simulink model "Satellte_Communications_System_TDMA"  (R2019b)
settings: Solver=ode45  StartTime=0.0  StopTime=inf  RelTol=1e-3  EnableMultiTasking=on
undefined symbols (not defined in the file): magnitude
libraries: dspstat3 x8, rfmathmodels1 x5, commrflib2 x4, commdigbbndpm3 x4, commfilt2 x4, dspsigattribs x4, dspmathops x4, dsparch4 x3, commrandsrc2 x2, commcnvcod2 x2, commsink2 x2, commutil2 x2
settings Model: Creator=123  LastModifiedBy=Steve
settings DataIOCC: LimitDataPoints=on  SaveFormat=Array  ReturnWorkspaceOutputs=off
settings OptimizationCC: LifeSpan=inf
settings DebuggingCC: SolverPrmCheckMsg=warning  SFUnexpectedBacktrackingDiag=warning  SFNoUnconditionalDefaultTransitionDiag=warning  SFExecutionAtInitializationDiag=none  ArithmeticOperatorsInVariantConditions=warning
settings HardwareCC: ProdBitPerPointer=32  ProdBitPerSizeT=32  ProdBitPerPtrDiffT=32  ProdLargestAtomicFloat=None  ProdIntDivRoundTo=Undefined  ProdEndianess=Unspecified  ProdWordSize=32  ProdHWDeviceType=32-bit Generic
settings ModelReferenceCC: PropagateSignalLabelsOutOfModel=off
settings SFSimCC: SimUseLocalCustomCode=off  CustomCodeUndefinedFunction=UseInterfaceOnly
settings RTWCC: RTWUseLocalCustomCode=off
settings CodeAppCC: StateflowObjectComments=on
settings GRTTargetCC: TargetLangStandard=C89/C90 (ANSI)  GeneratePreprocessorConditionals=Disable all
settings ConfigComp: CovMetricSettings=dw  CovHtmlReporting=on  CovSaveCumulativeToWorkspaceVar=on  CovSaveSingleToWorkspaceVar=on  CovExternalEMLEnable=off  CovSFcnEnable=off

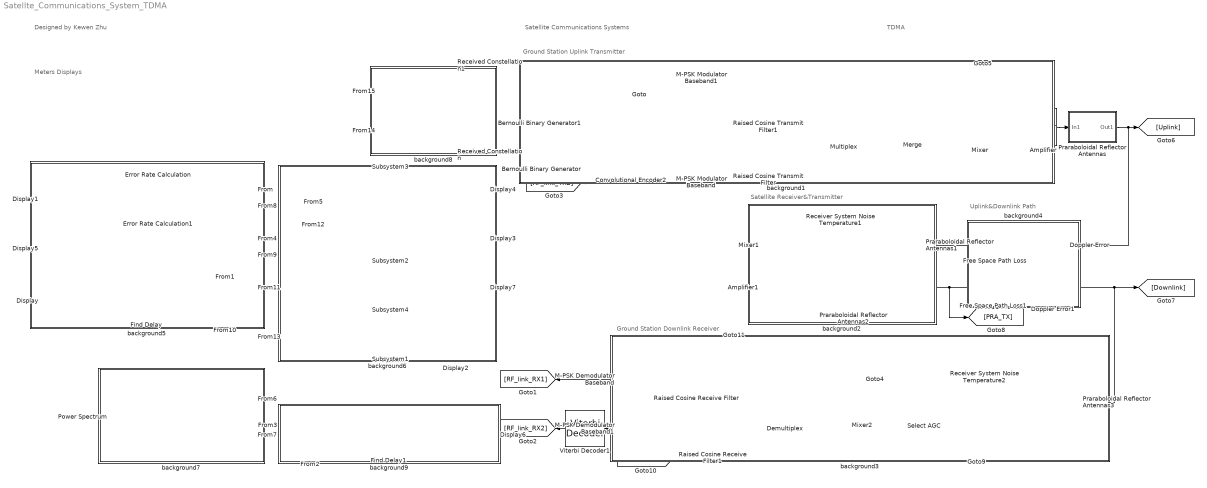
== system Satellte_Communications_System_TDMA ==
  note: Satellite Communications Systems
  note: Ground Station Uplink Transmitter
  note: Satellite Receiver&Transmitter
  note: Ground Station Downlink Receiver
  note: Uplink&Downlink Path
  note: Meters Displays
  note: Designed by Kewen Zhu
  note: TDMA
  Amplifier : rfmathmodels1/Amplifier  model_select=Saleh model  linGaindB=70  GindB=-21  iip3=30  am2pm=10  PwrAMPMStart=10  PwrAMPMEnd=inf  amam=[2.1587 1.1517]  ampm=[4.0033 9.1040]  x=[8.1081 1.5413 6.5202 -0.0718]  y=[4.6645 2.0965 10.88 -0.003]  p=0.5  GoutdB=70  vsat=1  method_select=Noise temperature  ntemp=0  nfigure=3.01  nfactor=2  seed=67987
      settings: SourceProductName=RF Blockset  SourceProductBaseCode=RB
  Amplifier1 : rfmathmodels1/Amplifier  model_select=Saleh model  linGaindB=84  GindB=-21  iip3=30  am2pm=10  PwrAMPMStart=10  PwrAMPMEnd=inf  amam=[2.1587 1.1517]  ampm=[4.0033 9.1040]  x=[8.1081 1.5413 6.5202 -0.0718]  y=[4.6645 2.0965 10.88 -0.003]  p=0.5  GoutdB=70  vsat=1  method_select=Noise temperature  ntemp=0  nfigure=3.01  nfactor=2  seed=67987
      settings: SourceProductName=RF Blockset  SourceProductBaseCode=RB
  Bernoulli Binary Generator : commrandsrc2/Bernoulli Binary Generator  P=0.5  seed=61  Ts=1/32000  frameBased=on  sampPerFrame=5100  orient=off  outDataType=double
      settings: SourceProductName=Communications Toolbox  SourceProductBaseCode=CM
  Bernoulli Binary Generator1 : commrandsrc2/Bernoulli Binary Generator  P=0.5  seed=61  Ts=1/64000  frameBased=on  sampPerFrame=10200  orient=off  outDataType=double
      settings: SourceProductName=Communications Toolbox  SourceProductBaseCode=CM
  Convolutional Encoder2 : commcnvcod2/Convolutional Encoder  trellis=poly2trellis(7, [171 133])  opMode=Continuous  DelayedResetAction=off  hasIniStPort=off  hasFinStPort=off  usePuncVector=off  punctureVector=[1; 1; 0; 1; 0; 1]  reset=Unused parameter value
      settings: SourceProductName=Communications Toolbox  SourceProductBaseCode=CM
  Demultiplex : Subsystem
  Display{,1..7} (8 alike) : Display
  Doppler Error : commrflib2/Phase// Frequency Offset  phaseOffset=0  freqPort=off  freqOffset=paramRFSatLink.DoppOffset
      settings: SourceProductName=Communications Toolbox
  Doppler Error1 : commrflib2/Phase// Frequency Offset  phaseOffset=0  freqPort=off  freqOffset=paramRFSatLink.DoppOffset
      settings: SourceProductName=Communications Toolbox
  Error Rate Calculation : commsink2/Error Rate Calculation  N=16  st_delay=0  cp_mode=Entire frame  subframe=[]  PMode=Port  WsName=ErrorVec  RsMode2=off  stop=off  numErr=100  maxBits=1e6
      settings: SourceProductName=Communications Toolbox
  Error Rate Calculation1 : commsink2/Error Rate Calculation  N=42  st_delay=0  cp_mode=Entire frame  subframe=[]  PMode=Port  WsName=ErrorVec  RsMode2=off  stop=off  numErr=100  maxBits=1e6
      settings: SourceProductName=Communications Toolbox
  Find Delay : commutil2/Find Delay  corrLength=200  chgSigOP=off  stopUpdate=off  numConstDelay=3
      settings: SourceProductName=Communications Toolbox  SourceProductBaseCode=CM
  Find Delay1 : commutil2/Find Delay  corrLength=200  chgSigOP=off  stopUpdate=off  numConstDelay=3
      settings: SourceProductName=Communications Toolbox  SourceProductBaseCode=CM
  Free Space Path Loss : commrflib2/Free Space Path Loss  mode=Distance and Frequency  dB=199  d=36000  fc=6000
      settings: SourceProductName=Communications Toolbox  SourceProductBaseCode=CM
  Free Space Path Loss1 : commrflib2/Free Space Path Loss  mode=Distance and Frequency  dB=196  d=36000  fc=4000
      settings: SourceProductName=Communications Toolbox  SourceProductBaseCode=CM
  M-PSK Demodulator Baseband : commdigbbndpm3/M-PSK Demodulator Baseband  M=4  OutType=Bit  DecType=Hard decision  VarSource=Dialog  Variance=1  Dec=Gray  Mapping=[0:7]  Ph=pi/4  outDtype1=Inherit via internal rule  outDtype2=Inherit via internal rule  derotateFactorWordLen=16  derotateFactorDataTypeStr=Inherit: Same word length as input  derotateFactorLastDataTypeStr=Inherit: Same word length as input
      settings: SourceProductName=Communications Toolbox
  M-PSK Demodulator Baseband1 : commdigbbndpm3/M-PSK Demodulator Baseband  M=4  OutType=Bit  DecType=Hard decision  VarSource=Dialog  Variance=1  Dec=Gray  Mapping=[0:7]  Ph=pi/4  outDtype1=Inherit via internal rule  outDtype2=Inherit via internal rule  derotateFactorWordLen=16  derotateFactorDataTypeStr=Inherit: Same word length as input  derotateFactorLastDataTypeStr=Inherit: Same word length as input
      settings: SourceProductName=Communications Toolbox
  M-PSK Modulator Baseband : commdigbbndpm3/M-PSK Modulator Baseband  M=4  InType=Bit  Enc=Gray  Mapping=[0:7]  Ph=pi/4  outDtype=double  outWordLen=16  outUDDataType=sfix(16)  outFracLenMode=Best precision  outFracLen=15  outDataTypeStr=double  outLastDataTypeStr=double
      settings: SourceProductName=Communications Toolbox
  M-PSK Modulator Baseband1 : commdigbbndpm3/M-PSK Modulator Baseband  M=4  InType=Bit  Enc=Gray  Mapping=[0:7]  Ph=pi/4  outDtype=double  outWordLen=16  outUDDataType=sfix(16)  outFracLenMode=Best precision  outFracLen=15  outDataTypeStr=double  outLastDataTypeStr=double
      settings: SourceProductName=Communications Toolbox
  Merge : Merge
  Mixer : rfmathmodels1/Mixer  gain=0  PhNs=-500  Fo=4e9  seed=2137  loss=0
      settings: SourceProductName=RF Blockset  SourceProductBaseCode=RB
  Mixer1 : rfmathmodels1/Mixer  gain=0  PhNs=-500  Fo=4e9  seed=2137  loss=0
      settings: SourceProductName=RF Blockset  SourceProductBaseCode=RB
  Mixer2 : rfmathmodels1/Mixer  gain=0  PhNs=-500  Fo=6e9  seed=2137  loss=0
      settings: SourceProductName=RF Blockset  SourceProductBaseCode=RB
  Multiplex : Subsystem
  Power Spectrum : Subsystem  TreatAsAtomicUnit=on
      mask Display: disp('Power\nSpectrum')
  Praraboloidal Reflector Antennas : Subsystem  mask(RF Transmit Antennas){f=6, D=15, g=0.6}
      mask prompts: f "Transmit Frequency(GHz)"; D "Antennas Caliber/Diameter(m)"; g "Gain factor(less than 1)"
      mask help:
      | Based on the Paraboloidal Reflector Antennas formula ,Gain factor is
      | G=(pi*D*f/c).^2*g
      mask init:
      | if isempty(f|D|g)
      |   gain= 0;
      |   s  = ['dB Gain'];
      | else
      |   f=f*10.^9;w=(3*10.^8)/f;
      |   G=(((pi*D/w).^2)*g).^0.5; 
      |   temp=((pi*D/w).^2)*g;
      |   gain=10*log10(temp);
      |   if (isscalar(f|D|g))
      |     s = sprintf('%g dB\n(%g)',gain,temp);
      |   else
      |     s = ['dB Gain'];
      |   end
      | end
      mask Display: fprintf(s)
  Praraboloidal Reflector Antennas1 : Subsystem  mask(RF Transmit Antennas){f=6, D=0.14, g=0.7}
      mask prompts: f "Transmit Frequency(GHz)"; D "Antennas Caliber/Diameter(m)"; g "Gain factor(less than 1)"
      mask help:
      | Based on the Paraboloidal Reflector Antennas formula ,Gain factor is
      | G=(pi*D*f/c).^2*g
      mask init: same as Satellte_Communications_System_TDMA/Praraboloidal Reflector Antennas
      mask Display: fprintf(s)
  Praraboloidal Reflector Antennas2 : Subsystem  mask(RF Transmit Antennas){f=4, D=0.4, g=0.7}
      mask prompts: f "Transmit Frequency(GHz)"; D "Antennas Caliber/Diameter(m)"; g "Gain factor(less than 1)"
      mask help:
      | Based on the Paraboloidal Reflector Antennas formula ,Gain factor is
      | G=(pi*D*f/c).^2*g
      mask init: same as Satellte_Communications_System_TDMA/Praraboloidal Reflector Antennas
      mask Display: fprintf(s)
  Praraboloidal Reflector Antennas3 : Subsystem  mask(RF Transmit Antennas){f=4, D=4.5, g=0.82}
      mask prompts: f "Transmit Frequency(GHz)"; D "Antennas Caliber/Diameter(m)"; g "Gain factor(less than 1)"
      mask help:
      | Based on the Paraboloidal Reflector Antennas formula ,Gain factor is
      | G=(pi*D*f/c).^2*g
      mask init: same as Satellte_Communications_System_TDMA/Praraboloidal Reflector Antennas
      mask Display: fprintf(s)
  Raised Cosine Receive Filter : commfilt2/Raised Cosine Receive Filter  filtType=Square root  R=0.2  filtSpan=8  N=8  downFactor=8  downOffset=0  filterGain=1  InputProcessing=Columns as channels (frame based)  RateOptions=Enforce single-rate processing  framing=Mute  checkCoeff=off  variableName=rcRxFilt  currentFiltSpan=8  D=(8)/2  inputOffset=0  sampMode=Mute  saveAsFlag=0  rateMode=Downsampling  checkGain=Normalized  launchFVT=on  roundingMode=Floor  overflowMode=off  coeffDataTypeStr=Inherit: Same word length as input  coeffMin=[]  coeffMax=[]  coeffLastDataTypeStr=Inherit: Same word length as input  accumDataTypeStr=Inherit: Same as product output  accumLastDataTypeStr=Inherit: Same as product output  outputDataTypeStr=Inherit: Same as accumulator  outputMin=[]  outputMax=[]  outputLastDataTypeStr=Inherit: Same as accumulator
      settings: SourceProductName=Communications Toolbox
  Raised Cosine Receive Filter1 : commfilt2/Raised Cosine Receive Filter  filtType=Square root  R=0.2  filtSpan=8  N=8  downFactor=8  downOffset=0  filterGain=1  InputProcessing=Columns as channels (frame based)  RateOptions=Enforce single-rate processing  framing=Mute  checkCoeff=off  variableName=rcRxFilt1  currentFiltSpan=8  D=(8)/2  inputOffset=0  sampMode=Mute  saveAsFlag=0  rateMode=Downsampling  checkGain=Normalized  launchFVT=on  roundingMode=Floor  overflowMode=off  coeffDataTypeStr=Inherit: Same word length as input  coeffMin=[]  coeffMax=[]  coeffLastDataTypeStr=Inherit: Same word length as input  accumDataTypeStr=Inherit: Same as product output  accumLastDataTypeStr=Inherit: Same as product output  outputDataTypeStr=Inherit: Same as accumulator  outputMin=[]  outputMax=[]  outputLastDataTypeStr=Inherit: Same as accumulator
      settings: SourceProductName=Communications Toolbox
  Raised Cosine Transmit Filter : commfilt2/Raised Cosine Transmit Filter  filtType=Square root  R=0.2  filtSpan=8  N=8  filterGain=1  InputProcessing=Columns as channels (frame based)  RateOptions=Enforce single-rate processing  framing=Mute  checkCoeff=off  variableName=rcTxFilt  checkGain=Normalized  sampMode=Mute  saveAsFlag=0  currentFiltSpan=8  D=(8)/2  launchFVT=on  roundingMode=Floor  overflowMode=off  coeffDataTypeStr=Inherit: Same word length as input  coeffMin=[]  coeffMax=[]  coeffLastDataTypeStr=Inherit: Same word length as input  outputDataTypeStr=Inherit: Same as accumulator  outputMin=[]  outputMax=[]  outputLastDataTypeStr=Inherit: Same as accumulator
      settings: SourceProductName=Communications Toolbox
  Raised Cosine Transmit Filter1 : commfilt2/Raised Cosine Transmit Filter  filtType=Square root  R=0.2  filtSpan=8  N=8  filterGain=1  InputProcessing=Columns as channels (frame based)  RateOptions=Enforce single-rate processing  framing=Mute  checkCoeff=off  variableName=rcTxFilt1  checkGain=Normalized  sampMode=Mute  saveAsFlag=0  currentFiltSpan=8  D=(8)/2  launchFVT=on  roundingMode=Floor  overflowMode=off  coeffDataTypeStr=Inherit: Same word length as input  coeffMin=[]  coeffMax=[]  coeffLastDataTypeStr=Inherit: Same word length as input  outputDataTypeStr=Inherit: Same as accumulator  outputMin=[]  outputMax=[]  outputLastDataTypeStr=Inherit: Same as accumulator
      settings: SourceProductName=Communications Toolbox
  Received Constellation : ConstellationDiagram  Tag=ScatterPlot
  Received Constellation1 : ConstellationDiagram  Tag=ScatterPlot
  Receiver System Noise Temperature1 : Subsystem  AncestorBlock=xd/RF/Receiver System Noise Temperature  TreatAsAtomicUnit=on  mask{T_sk=10, T_su=300, Eff=0.72, Te=250, Seed=123456789}
      mask prompts: T_sk "Sky Temperature(K):"; T_su "Surface Temperature(K):"; Eff "Beam Efficiency(less than 1):"; Te "The Noise Temperature of Receiver Facility(K):"; Seed "Initial seed"
      mask init:
      | Ta=T_sk*Eff+T_sk*(1-Eff)*0.5...
      |     +T_su*0.5*(1-Eff);
      | T_all=Ta+Te;
      | str = ['Noise\nTemperature\n' num2str(T_all) ' K'];
      mask Display: disp(str);
  Receiver System Noise Temperature2 : Subsystem  AncestorBlock=xd/RF/Receiver System Noise Temperature  TreatAsAtomicUnit=on  mask{T_sk=10, T_su=300, Eff=0.72, Te=100, Seed=123456789}
      mask prompts: T_sk "Sky Temperature(K):"; T_su "Surface Temperature(K):"; Eff "Beam Efficiency(less than 1):"; Te "The Noise Temperature of Receiver Facility(K):"; Seed "Initial seed"
      mask init:
      | Ta=T_sk*Eff+T_sk*(1-Eff)*0.5...
      |     +T_su*0.5*(1-Eff);
      | T_all=Ta+Te;
      | str = ['Noise\nTemperature\n' num2str(T_all) ' K'];
      mask Display: disp(str);
  Select AGC : Subsystem  mask{swCase=Magnitude}
      mask prompts: swCase "Case Value:"
      mask init:
      | charCase = char(swCase);
      | switch charCase,
      | case 'I and Q',
      | 		selValue = 1;
      | otherwise,
      | 		selValue = 0;
      | end
      mask TypeOptions swCase: Magnitude | I and Q
      mask Display: disp([char(swCase) '\nAGC'])
  Subsystem1 : Subsystem
      mask Display: disp('Test Power')
  Subsystem2 : Subsystem
      mask Display: disp('Test Power')
  Subsystem3 : Subsystem
      mask Display: disp('Test Power')
  Subsystem4 : Subsystem
      mask Display: disp('Test Power')
  Viterbi Decoder1 : commcnvcod2/Viterbi Decoder  trellis=poly2trellis(7, [171 133])  isPunctured=off  punctureVector=[1; 1; 0; 1; 0; 1]  erasures=off  dectype=Hard decision  nsdecb=4  runSigValErrCheck=off  tbdepth=34  opmode=Continuous  reset=off  delayedResetAction=off  smWordLength=16  outDataType=double
      settings: SourceProductName=Communications Toolbox  SourceProductBaseCode=CM
  background1 : Subsystem
      mask Display: disp('')
  background2 : Subsystem
      mask Display: disp('')
  background3 : Subsystem
      mask Display: disp('')
  background4 : Subsystem
      mask Display: disp('')
  background5 : Subsystem
      mask Display: disp('')
  background6 : Subsystem
      mask Display: disp('')
  background7 : Subsystem
      mask Display: disp('')
  background8 : Subsystem
      mask Display: disp('')
  background9 : Subsystem
      mask Display: disp('')
  wires:
  M-PSK Modulator Baseband/1 -> Raised Cosine Transmit Filter/1
  Praraboloidal Reflector Antennas/1(Out1) -> [Uplink], Doppler Error/1
  Free Space Path Loss/1 -> Praraboloidal Reflector Antennas1/1(In1)
  Praraboloidal Reflector Antennas1/1(Out1) -> Receiver System Noise Temperature1/1(In1)
  Mixer/1 -> Amplifier/1
  Receiver System Noise Temperature1/1(Out1) -> Mixer1/1
  Praraboloidal Reflector Antennas2/1(Out1) -> [PRA_TX], Free Space Path Loss1/1
  Subsystem2/1(Out2) -> Display3/1
  Free Space Path Loss1/1 -> Doppler Error1/1
  Praraboloidal Reflector Antennas3/1(Out1) -> [PRA_RX], Receiver System Noise Temperature2/1(In1)
  Receiver System Noise Temperature2/1(Out1) -> Select AGC/1(In2)
  Select AGC/1(Out1) -> Mixer2/1
  Mixer2/1 -> Demultiplex/2(In2), Demultiplex/1(In1), [RX_FDMA]
  Subsystem1/1(Out2) -> Display2/1
  Error Rate Calculation/1 -> Display1/1
  Find Delay/1 -> Display/1
  Subsystem3/1(Out2) -> Display4/1
  M-PSK Modulator Baseband1/1 -> Raised Cosine Transmit Filter1/1
  Raised Cosine Transmit Filter/1 -> Multiplex/2(In2)
  Raised Cosine Transmit Filter1/1 -> Multiplex/1(In1)
  Amplifier/1 -> Praraboloidal Reflector Antennas/1(In1)
  Demultiplex/2(Out2) -> Raised Cosine Receive Filter1/1
  Demultiplex/1(Out1) -> Raised Cosine Receive Filter/1
  Error Rate Calculation1/1 -> Display5/1
  Find Delay1/1 -> Display6/1
  Bernoulli Binary Generator1/1 -> [RF_link_TX1], M-PSK Modulator Baseband1/1
  Bernoulli Binary Generator/1 -> [RF_link_TX2], Convolutional Encoder2/1
  Convolutional Encoder2/1 -> M-PSK Modulator Baseband/1
  Raised Cosine Receive Filter/1 -> [RX1_const], M-PSK Demodulator Baseband/1
  Raised Cosine Receive Filter1/1 -> [RX2_const], M-PSK Demodulator Baseband1/1
  M-PSK Demodulator Baseband1/1 -> Viterbi Decoder1/1
  Merge/1 -> [TX_FDMA], Mixer/1
  Amplifier1/1 -> Praraboloidal Reflector Antennas2/1(In1)
  Mixer1/1 -> Amplifier1/1
  Doppler Error1/1 -> [Downlink], Praraboloidal Reflector Antennas3/1(In1)
  Doppler Error/1 -> Free Space Path Loss/1
  [RF_link_TX1] -> Error Rate Calculation/1
  [RF_link_TX1] -> Find Delay/1
  [RF_link_TX2] -> Find Delay1/1
  [RF_link_TX2] -> Error Rate Calculation1/1
  Viterbi Decoder1/1 -> [RF_link_RX2]
  [RF_link_RX2] -> Error Rate Calculation1/2
  [RF_link_TX1] -> Find Delay1/2
  M-PSK Demodulator Baseband/1 -> [RF_link_RX1]
  [RF_link_RX1] -> Error Rate Calculation/2
  [RF_link_RX1] -> Find Delay/2
  [RX_FDMA] -> Power Spectrum/2(In2)
  [TX_FDMA] -> Power Spectrum/1(In1)
  Subsystem4/1(Out2) -> Display7/1
  [Uplink] -> Subsystem3/1(In1)
  [Downlink] -> Subsystem4/1(In1)
  [PRA_TX] -> Subsystem2/1(In1)
  [PRA_RX] -> Subsystem1/1(In1)
  [RX2_const] -> Received Constellation/1
  [RX1_const] -> Received Constellation1/1
  Multiplex/1(Out1) -> Merge/1
  Multiplex/2(Out2) -> Merge/2

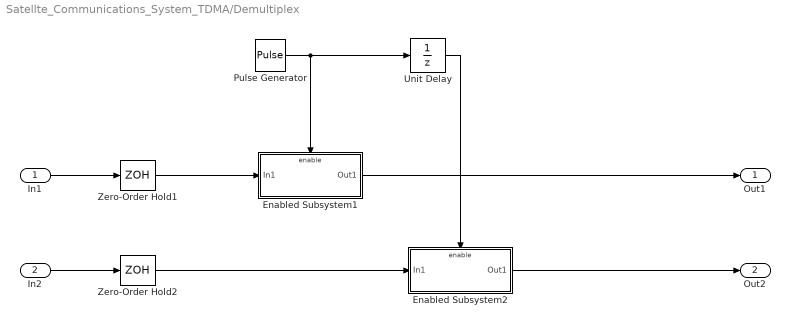
== system Satellte_Communications_System_TDMA/Demultiplex ==
  In1 : Inport
  In2 : Inport  Port=2
  Enabled Subsystem1 : Subsystem  TreatAsAtomicUnit=on
  Enabled Subsystem2 : Subsystem  TreatAsAtomicUnit=on
  Pulse Generator : DiscretePulseGenerator  Period=3  SampleTime=0.001
  Unit Delay : UnitDelay  SampleTime=0.001
  Zero-Order Hold1 : ZeroOrderHold  SampleTime=0.001
  Zero-Order Hold2 : ZeroOrderHold  SampleTime=0.001
  Out1 : Outport
  Out2 : Outport  Port=2
  wires:
  In1/1 -> Zero-Order Hold1/1
  In2/1 -> Zero-Order Hold2/1
  Zero-Order Hold1/1 -> Enabled Subsystem1/1(In1)
  Pulse Generator/1 -> Unit Delay/1, Enabled Subsystem1/Enable
  Enabled Subsystem1/1(Out1) -> Out1/1
  Zero-Order Hold2/1 -> Enabled Subsystem2/1(In1)
  Unit Delay/1 -> Enabled Subsystem2/Enable
  Enabled Subsystem2/1(Out1) -> Out2/1

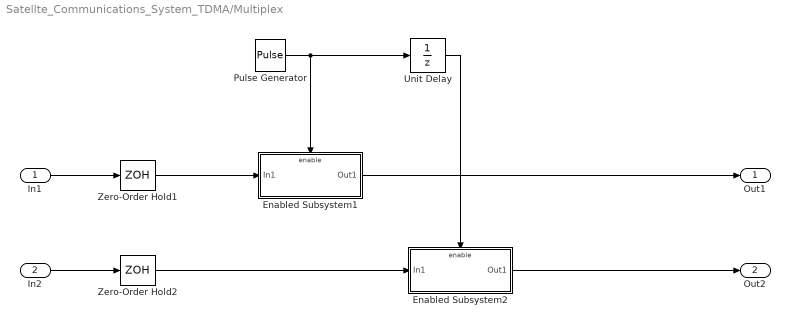
== system Satellte_Communications_System_TDMA/Multiplex ==
  In1 : Inport
  In2 : Inport  Port=2
  Enabled Subsystem1 : Subsystem  TreatAsAtomicUnit=on
  Enabled Subsystem2 : Subsystem  TreatAsAtomicUnit=on
  Pulse Generator : DiscretePulseGenerator  Period=3  SampleTime=0.001
  Unit Delay : UnitDelay  SampleTime=0.001
  Zero-Order Hold1 : ZeroOrderHold  SampleTime=0.001
  Zero-Order Hold2 : ZeroOrderHold  SampleTime=0.001
  Out1 : Outport
  Out2 : Outport  Port=2
  wires:
  In1/1 -> Zero-Order Hold1/1
  In2/1 -> Zero-Order Hold2/1
  Zero-Order Hold1/1 -> Enabled Subsystem1/1(In1)
  Pulse Generator/1 -> Unit Delay/1, Enabled Subsystem1/Enable
  Enabled Subsystem1/1(Out1) -> Out1/1
  Zero-Order Hold2/1 -> Enabled Subsystem2/1(In1)
  Unit Delay/1 -> Enabled Subsystem2/Enable
  Enabled Subsystem2/1(Out1) -> Out2/1

== system Satellte_Communications_System_TDMA/Power Spectrum ==
  In1 : Inport
  In2 : Inport  Port=2
  Matrix Concatenation : Concatenate  Mode=Multidimensional array  ConcatenateDimension=2
  Tx and Rx Spectrum : SpectrumAnalyzer
      settings: AttributesFormatString=\n
  wires:
  In1/1 -> Matrix Concatenation/1
  In2/1 -> Matrix Concatenation/2
  Matrix Concatenation/1 -> Tx and Rx Spectrum/1

== system Satellte_Communications_System_TDMA/Praraboloidal Reflector Antennas ==
  In1 : Inport
  Gain : Gain  Gain=G
  Out1 : Outport
  wires:
  Gain/1 -> Out1/1
  In1/1 -> Gain/1

== system Satellte_Communications_System_TDMA/Praraboloidal Reflector Antennas1 ==
  In1 : Inport
  Gain : Gain  Gain=G
  Out1 : Outport
  wires:
  Gain/1 -> Out1/1
  In1/1 -> Gain/1

== system Satellte_Communications_System_TDMA/Praraboloidal Reflector Antennas2 ==
  In1 : Inport
  Gain : Gain  Gain=G
  Out1 : Outport
  wires:
  Gain/1 -> Out1/1
  In1/1 -> Gain/1

== system Satellte_Communications_System_TDMA/Praraboloidal Reflector Antennas3 ==
  In1 : Inport
  Gain : Gain  Gain=G
  Out1 : Outport
  wires:
  Gain/1 -> Out1/1
  In1/1 -> Gain/1

== system Satellte_Communications_System_TDMA/Receiver System Noise Temperature1 ==
  In1 : Inport
  Receiver Thermal Noise : Subsystem  AncestorBlock=commrflib2/Receiver Thermal Noise  mask(Receiver Thermal Noise){method=Noise temperature, ntemp=T_all, nfigure=3.01, nfactor=2, seed=Seed}
      mask prompts: method "Specification method:"; ntemp "Noise temperature (K):"; nfigure "Noise figure (dB):"; nfactor "Noise factor:"; seed "Initial seed:"
      mask help:
      | Complex baseband model of receiver thermal noise.
      |
      | The amount of noise added to the input signal may be specified either in terms of noise temperature, noise figure, or noise factor.
      mask init:
      | k=1.380650e-23; % Boltzmann's constant, J/K
      | 
      | switch method
      | case 'Noise temperature',
      | 	T = ntemp;
      | 	str = ['Noise\nTemperature\n' num2str(ntemp) ' K'];
      | case 'Noise figure',
      | 	nfactor = 10.^(0.1*nfigure);
      | 	T = 290*(nfactor-1);
      | 	str = ['Noise\nFigure\n' num2str(nfigure) ' dB'];
      | case 'Noise factor',
      | 	T = 290*(nfactor-1);
      | 	str = ['Noise\nFactor\n' num2str(nfactor)];
      | end
      | 
      | kT=k*T;
      mask Help: helpview(commbhelp)
      mask TypeOptions method: Noise temperature | Noise figure | Noise factor
      mask Callback method:
      | switch get_param(gcb,'method')
      | 
      | case 'Noise temperature',
      | 
      | 	set_param(gcb,'maskvisibilities',{'on' 'on' 'off' 'off' 'on'},...
      |         'maskenables',{'on' 'on' 'off' 'off' 'on'});
      | 
      | case 'Noise figure',
      | 
      | 	set_param(gcb,'maskvisibilities',{'on' 'off' 'on' 'off' 'on'},...
      |     'maskenables',{'on' 'off' 'on' 'off' 'on'});
      | 
      | case 'Noise factor',
      | 
      | 	set_param(gcb,'maskvisibilities',{'on' 'off' 'off' 'on' 'on'},...
      |         'maskenables',{'on' 'off' 'off' 'on' 'on'});
      | 
      | end
      mask Display: disp(str);
  Out1 : Outport
  wires:
  Receiver Thermal Noise/1(Out1) -> Out1/1
  In1/1 -> Receiver Thermal Noise/1(In1)

== system Satellte_Communications_System_TDMA/Receiver System Noise Temperature2 ==
  In1 : Inport
  Receiver Thermal Noise : Subsystem  AncestorBlock=commrflib2/Receiver Thermal Noise  mask(Receiver Thermal Noise){method=Noise temperature, ntemp=T_all, nfigure=3.01, nfactor=2, seed=Seed}
      mask prompts: method "Specification method:"; ntemp "Noise temperature (K):"; nfigure "Noise figure (dB):"; nfactor "Noise factor:"; seed "Initial seed:"
      mask help:
      | Complex baseband model of receiver thermal noise.
      |
      | The amount of noise added to the input signal may be specified either in terms of noise temperature, noise figure, or noise factor.
      mask init: same as Satellte_Communications_System_TDMA/Receiver System Noise Temperature1/Receiver Thermal Noise
      mask Help: helpview(commbhelp)
      mask TypeOptions method: Noise temperature | Noise figure | Noise factor
      mask Callback method:
      | switch get_param(gcb,'method')
      | 
      | case 'Noise temperature',
      | 
      | 	set_param(gcb,'maskvisibilities',{'on' 'on' 'off' 'off' 'on'},...
      |         'maskenables',{'on' 'on' 'off' 'off' 'on'});
      | 
      | case 'Noise figure',
      | 
      | 	set_param(gcb,'maskvisibilities',{'on' 'off' 'on' 'off' 'on'},...
      |     'maskenables',{'on' 'off' 'on' 'off' 'on'});
      | 
      | case 'Noise factor',
      | 
      | 	set_param(gcb,'maskvisibilities',{'on' 'off' 'off' 'on' 'on'},...
      |         'maskenables',{'on' 'off' 'off' 'on' 'on'});
      | 
      | end
      mask Display: disp(str);
  Out1 : Outport
  wires:
  Receiver Thermal Noise/1(Out1) -> Out1/1
  In1/1 -> Receiver Thermal Noise/1(In1)

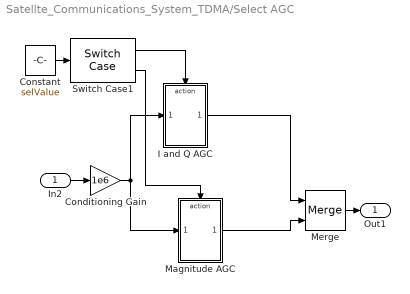
== system Satellte_Communications_System_TDMA/Select AGC ==
  In2 : Inport
  Conditioning Gain : Gain  Gain=1e6  SaturateOnIntegerOverflow=on  OutDataTypeStr=Inherit: Same as input  ParamDataTypeStr=Inherit: Same as input
  Constant : Constant  Value=selValue
  I and Q AGC : Subsystem  TreatAsAtomicUnit=on
  Magnitude AGC : Subsystem  TreatAsAtomicUnit=on
  Merge : Merge  InitialOutput=0
  Switch Case1 : SwitchCase
  Out1 : Outport
  wires:
  Switch Case1/2 -> Magnitude AGC/Action
  Switch Case1/1 -> I and Q AGC/Action
  Constant/1 -> Switch Case1/1
  In2/1 -> Conditioning Gain/1
  I and Q AGC/1(Out1) -> Merge/1
  Magnitude AGC/1(Out1) -> Merge/2
  Merge/1 -> Out1/1
  Conditioning Gain/1 -> I and Q AGC/1(In1), Magnitude AGC/1(In1)

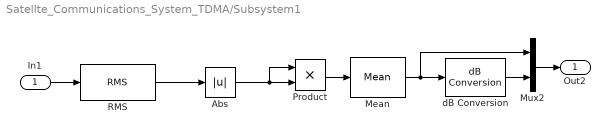
== system Satellte_Communications_System_TDMA/Subsystem1 ==
  In1 : Inport
  Abs : Abs
  Mean : dspstat3/Mean  run=off  InputProcessing=Columns as channels (frame based)  reset_popup=None  directionMode=Entire input  dimension=1  roiEnable=off  roiType=Rectangles  roiPortion=Entire ROI  roiOutput=Individual statistics for each ROI  roiFlag=off  roundingMode=Floor  overflowMode=off  outputDataTypeStr=Inherit: Same as accumulator  outputMin=[]  outputMax=[]  outputLastDataTypeStr=Inherit: Same as accumulator
  Mux2 : Mux  Inputs=2
  Product : Product
  RMS : dspstat3/RMS  run=off  directionMode=Each column  dimension=1  InputProcessing=Columns as channels (frame based)  reset_popup=None
  dB Conversion : dspmathops/dB Conversion  dBtype=dB  intype=Power  R=1  fuzz=off
      settings: SourceProductName=DSP System Toolbox
  Out2 : Outport
  wires:
  Mux2/1 -> Out2/1
  Product/1 -> Mean/1
  Mean/1 -> Mux2/1, dB Conversion/1
  dB Conversion/1 -> Mux2/2
  Abs/1 -> Product/2, Product/1
  In1/1 -> RMS/1
  RMS/1 -> Abs/1

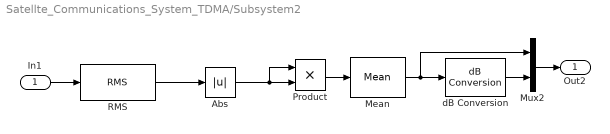
== system Satellte_Communications_System_TDMA/Subsystem2 ==
  In1 : Inport
  Abs : Abs
  Mean : dspstat3/Mean  run=off  InputProcessing=Columns as channels (frame based)  reset_popup=None  directionMode=Entire input  dimension=1  roiEnable=off  roiType=Rectangles  roiPortion=Entire ROI  roiOutput=Individual statistics for each ROI  roiFlag=off  roundingMode=Floor  overflowMode=off  outputDataTypeStr=Inherit: Same as accumulator  outputMin=[]  outputMax=[]  outputLastDataTypeStr=Inherit: Same as accumulator
  Mux2 : Mux  Inputs=2
  Product : Product
  RMS : dspstat3/RMS  run=off  directionMode=Each column  dimension=1  InputProcessing=Columns as channels (frame based)  reset_popup=None
  dB Conversion : dspmathops/dB Conversion  dBtype=dB  intype=Power  R=1  fuzz=off
      settings: SourceProductName=DSP System Toolbox
  Out2 : Outport
  wires:
  Mux2/1 -> Out2/1
  Product/1 -> Mean/1
  Mean/1 -> Mux2/1, dB Conversion/1
  dB Conversion/1 -> Mux2/2
  Abs/1 -> Product/2, Product/1
  In1/1 -> RMS/1
  RMS/1 -> Abs/1

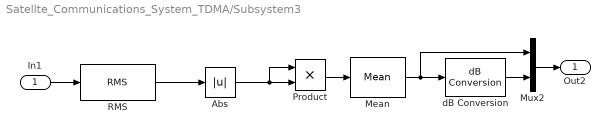
== system Satellte_Communications_System_TDMA/Subsystem3 ==
  In1 : Inport
  Abs : Abs
  Mean : dspstat3/Mean  run=off  InputProcessing=Columns as channels (frame based)  reset_popup=None  directionMode=Entire input  dimension=1  roiEnable=off  roiType=Rectangles  roiPortion=Entire ROI  roiOutput=Individual statistics for each ROI  roiFlag=off  roundingMode=Floor  overflowMode=off  outputDataTypeStr=Inherit: Same as accumulator  outputMin=[]  outputMax=[]  outputLastDataTypeStr=Inherit: Same as accumulator
  Mux2 : Mux  Inputs=2
  Product : Product
  RMS : dspstat3/RMS  run=off  directionMode=Each column  dimension=1  InputProcessing=Columns as channels (frame based)  reset_popup=None
  dB Conversion : dspmathops/dB Conversion  dBtype=dB  intype=Power  R=1  fuzz=off
      settings: SourceProductName=DSP System Toolbox
  Out2 : Outport
  wires:
  Mux2/1 -> Out2/1
  Product/1 -> Mean/1
  Mean/1 -> Mux2/1, dB Conversion/1
  dB Conversion/1 -> Mux2/2
  Abs/1 -> Product/2, Product/1
  In1/1 -> RMS/1
  RMS/1 -> Abs/1

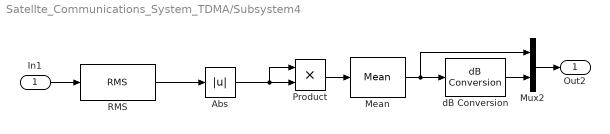
== system Satellte_Communications_System_TDMA/Subsystem4 ==
  In1 : Inport
  Abs : Abs
  Mean : dspstat3/Mean  run=off  InputProcessing=Columns as channels (frame based)  reset_popup=None  directionMode=Entire input  dimension=1  roiEnable=off  roiType=Rectangles  roiPortion=Entire ROI  roiOutput=Individual statistics for each ROI  roiFlag=off  roundingMode=Floor  overflowMode=off  outputDataTypeStr=Inherit: Same as accumulator  outputMin=[]  outputMax=[]  outputLastDataTypeStr=Inherit: Same as accumulator
  Mux2 : Mux  Inputs=2
  Product : Product
  RMS : dspstat3/RMS  run=off  directionMode=Each column  dimension=1  InputProcessing=Columns as channels (frame based)  reset_popup=None
  dB Conversion : dspmathops/dB Conversion  dBtype=dB  intype=Power  R=1  fuzz=off
      settings: SourceProductName=DSP System Toolbox
  Out2 : Outport
  wires:
  Mux2/1 -> Out2/1
  Product/1 -> Mean/1
  Mean/1 -> Mux2/1, dB Conversion/1
  dB Conversion/1 -> Mux2/2
  Abs/1 -> Product/2, Product/1
  In1/1 -> RMS/1
  RMS/1 -> Abs/1

== system Satellte_Communications_System_TDMA/background1 ==

== system Satellte_Communications_System_TDMA/background2 ==

== system Satellte_Communications_System_TDMA/background3 ==

== system Satellte_Communications_System_TDMA/background4 ==

== system Satellte_Communications_System_TDMA/background5 ==

== system Satellte_Communications_System_TDMA/background6 ==

== system Satellte_Communications_System_TDMA/background7 ==

== system Satellte_Communications_System_TDMA/background8 ==

== system Satellte_Communications_System_TDMA/background9 ==

== system Satellte_Communications_System_TDMA/Demultiplex/Enabled Subsystem1 ==
  In1 : Inport
  Enable : EnablePort
  Out1 : Outport
  wires:
  In1/1 -> Out1/1

== system Satellte_Communications_System_TDMA/Demultiplex/Enabled Subsystem2 ==
  In1 : Inport
  Enable : EnablePort
  Out1 : Outport
  wires:
  In1/1 -> Out1/1

== system Satellte_Communications_System_TDMA/Multiplex/Enabled Subsystem1 ==
  In1 : Inport
  Enable : EnablePort
  Out1 : Outport
  wires:
  In1/1 -> Out1/1

== system Satellte_Communications_System_TDMA/Multiplex/Enabled Subsystem2 ==
  In1 : Inport
  Enable : EnablePort
  Out1 : Outport
  wires:
  In1/1 -> Out1/1

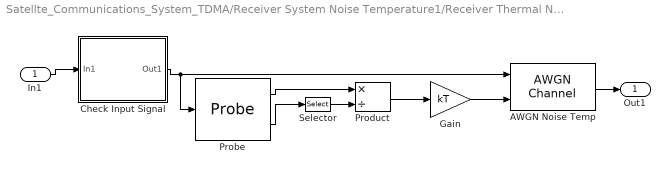
== system Satellte_Communications_System_TDMA/Receiver System Noise Temperature1/Receiver Thermal Noise ==
  In1 : Inport
  AWGN Noise Temp : commchan3/AWGN Channel  InputProcessing=Columns as channels (frame based)  seed=seed  noiseMode=Variance from port  EbNodB=10  EsNodB=10  SNRdB=10  bitsPerSym=1  Ps=1  Tsym=1  variance=var
      settings: SourceProductName=Communications Toolbox
  Check Input Signal : Subsystem
      mask Display: disp('Check\nInput Signal');
  Gain : Gain  Gain=kT  SaturateOnIntegerOverflow=on  OutDataTypeStr=Inherit: Same as input  ParamDataTypeStr=Inherit: Same as input
  Probe : Probe  ProbeComplexSignal=off  ProbeWidthDataType=Same as input  ProbeSampleTimeDataType=Same as input
  Product : Product  Inputs=*/  SaturateOnIntegerOverflow=on  InputSameDT=on  OutDataTypeStr=Inherit: Same as first input
  Selector : Selector  InputPortWidth=2  IndexOptions=Index vector (dialog)  Indices=1  OutputSizes=1
  Out1 : Outport
  wires:
  Check Input Signal/1(Out1) -> Probe/1, AWGN Noise Temp/1
  Selector/1 -> Product/2
  Probe/2 -> Selector/1
  Gain/1 -> AWGN Noise Temp/2
  Product/1 -> Gain/1
  Probe/1 -> Product/1
  In1/1 -> Check Input Signal/1(In1)
  AWGN Noise Temp/1 -> Out1/1

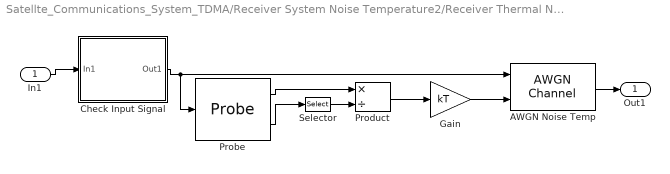
== system Satellte_Communications_System_TDMA/Receiver System Noise Temperature2/Receiver Thermal Noise ==
  In1 : Inport
  AWGN Noise Temp : commchan3/AWGN Channel  InputProcessing=Columns as channels (frame based)  seed=seed  noiseMode=Variance from port  EbNodB=10  EsNodB=10  SNRdB=10  bitsPerSym=1  Ps=1  Tsym=1  variance=var
      settings: SourceProductName=Communications Toolbox
  Check Input Signal : Subsystem
      mask Display: disp('Check\nInput Signal');
  Gain : Gain  Gain=kT  SaturateOnIntegerOverflow=on  OutDataTypeStr=Inherit: Same as input  ParamDataTypeStr=Inherit: Same as input
  Probe : Probe  ProbeComplexSignal=off  ProbeWidthDataType=Same as input  ProbeSampleTimeDataType=Same as input
  Product : Product  Inputs=*/  SaturateOnIntegerOverflow=on  InputSameDT=on  OutDataTypeStr=Inherit: Same as first input
  Selector : Selector  InputPortWidth=2  IndexOptions=Index vector (dialog)  Indices=1  OutputSizes=1
  Out1 : Outport
  wires:
  Check Input Signal/1(Out1) -> Probe/1, AWGN Noise Temp/1
  Selector/1 -> Product/2
  Probe/2 -> Selector/1
  Gain/1 -> AWGN Noise Temp/2
  Product/1 -> Gain/1
  Probe/1 -> Product/1
  In1/1 -> Check Input Signal/1(In1)
  AWGN Noise Temp/1 -> Out1/1

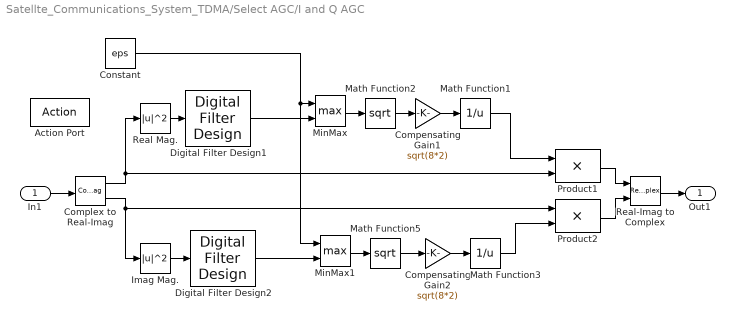
== system Satellte_Communications_System_TDMA/Select AGC/I and Q AGC ==
  In1 : Inport
  Action Port : ActionPort  PropagateVarSize=During execution  ActionPortLabel=case [ 1 ]:
  Compensating Gain1 : Gain  Gain=sqrt(8*2)  SaturateOnIntegerOverflow=on  OutDataTypeStr=Inherit: Same as input  ParamDataTypeStr=Inherit: Same as input
  Compensating Gain2 : Gain  Gain=sqrt(8*2)  SaturateOnIntegerOverflow=on  OutDataTypeStr=Inherit: Same as input  ParamDataTypeStr=Inherit: Same as input
  Complex to Real-Imag : ComplexToRealImag
  Constant : Constant  Value=eps  VectorParams1D=off  FramePeriod=-1
      settings: SamplingMode=Frame based
  Digital Filter Design1 : dsparch4/Digital Filter Design  mwdsp_browser_bugfix_var=off
  Digital Filter Design2 : dsparch4/Digital Filter Design  mwdsp_browser_bugfix_var=off
  Imag Mag. : Math  Operator=magnitude^2  SaturateOnIntegerOverflow=on
  Math Function1 : Math  Operator=reciprocal  SaturateOnIntegerOverflow=on
  Math Function2 : Math  Operator=sqrt  SaturateOnIntegerOverflow=on
  Math Function3 : Math  Operator=reciprocal  SaturateOnIntegerOverflow=on
  Math Function5 : Math  Operator=sqrt  SaturateOnIntegerOverflow=on
  MinMax : MinMax  Function=max  Inputs=2  SaturateOnIntegerOverflow=on  InputSameDT=on
  MinMax1 : MinMax  Function=max  Inputs=2  SaturateOnIntegerOverflow=on  InputSameDT=on
  Product1 : Product  SaturateOnIntegerOverflow=on  OutDataTypeStr=Inherit: Same as first input
  Product2 : Product  SaturateOnIntegerOverflow=on  OutDataTypeStr=Inherit: Same as first input
  Real Mag. : Math  Operator=magnitude^2  SaturateOnIntegerOverflow=on
  Real-Imag to Complex : RealImagToComplex
  Out1 : Outport
  wires:
  Real-Imag to Complex/1 -> Out1/1
  In1/1 -> Complex to Real-Imag/1
  Math Function3/1 -> Product2/2
  Math Function1/1 -> Product1/1
  Product2/1 -> Real-Imag to Complex/2
  Product1/1 -> Real-Imag to Complex/1
  Math Function5/1 -> Compensating Gain2/1
  Compensating Gain2/1 -> Math Function3/1
  Complex to Real-Imag/2 -> Product2/1, Imag Mag./1
  Complex to Real-Imag/1 -> Product1/2, Real Mag./1
  Imag Mag./1 -> Digital Filter Design2/1
  Real Mag./1 -> Digital Filter Design1/1
  Math Function2/1 -> Compensating Gain1/1
  Compensating Gain1/1 -> Math Function1/1
  Constant/1 -> MinMax/1, MinMax1/1
  Digital Filter Design1/1 -> MinMax/2
  Digital Filter Design2/1 -> MinMax1/2
  MinMax1/1 -> Math Function5/1
  MinMax/1 -> Math Function2/1

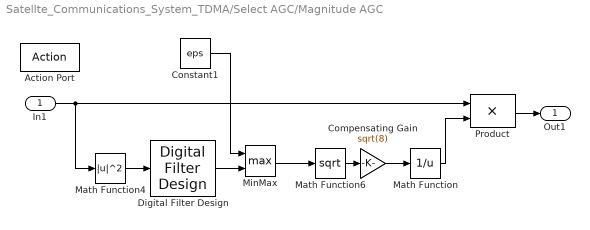
== system Satellte_Communications_System_TDMA/Select AGC/Magnitude AGC ==
  In1 : Inport
  Action Port : ActionPort  PropagateVarSize=During execution  ActionPortLabel=default:
  Compensating Gain : Gain  Gain=sqrt(8)  SaturateOnIntegerOverflow=on  OutDataTypeStr=Inherit: Same as input  ParamDataTypeStr=Inherit: Same as input
  Constant1 : Constant  Value=eps  VectorParams1D=off  FramePeriod=-1
      settings: SamplingMode=Frame based
  Digital Filter Design : dsparch4/Digital Filter Design  mwdsp_browser_bugfix_var=off
  Math Function : Math  Operator=reciprocal  SaturateOnIntegerOverflow=on
  Math Function4 : Math  Operator=magnitude^2  SaturateOnIntegerOverflow=on
  Math Function6 : Math  Operator=sqrt  SaturateOnIntegerOverflow=on
  MinMax : MinMax  Function=max  Inputs=2  SaturateOnIntegerOverflow=on  InputSameDT=on
  Product : Product  SaturateOnIntegerOverflow=on  OutDataTypeStr=Inherit: Same as first input
  Out1 : Outport
  wires:
  Product/1 -> Out1/1
  In1/1 -> Math Function4/1, Product/1
  Compensating Gain/1 -> Math Function/1
  Math Function6/1 -> Compensating Gain/1
  Math Function4/1 -> Digital Filter Design/1
  Math Function/1 -> Product/2
  Digital Filter Design/1 -> MinMax/2
  MinMax/1 -> Math Function6/1
  Constant1/1 -> MinMax/1

== system Satellte_Communications_System_TDMA/Receiver System Noise Temperature1/Receiver Thermal Noise/Check Input Signal ==
  In1 : Inport
  Check Signal Attributes : dspsigattribs/Check Signal Attributes  SigAttribCheckMethod=Does not match attributes exactly  Complexity=Complex  Frame=Ignore  DimsCheckMethod=Is...  Dimensions=Column vector (2-D) or scalar  DatatypeCheckMethod=Is...  DatatypeGeneral=Floating-point  DtypeFloatSpecific=Any floating-point  DtypeFixedSpecific=Any fixed-point  DtypeIntSpecific=Any integer  SampleMode=Ignore
      settings: SourceProductName=DSP System Toolbox  SourceProductBaseCode=DS
  Check Signal Attributes1 : dspsigattribs/Check Signal Attributes  SigAttribCheckMethod=Matches attributes exactly  Complexity=Ignore  Frame=Sample-based  DimsCheckMethod=Is...  Dimensions=Vector (1-D or 2-D)  DatatypeCheckMethod=Ignore  DatatypeGeneral=Boolean  DtypeFloatSpecific=Any floating-point  DtypeFixedSpecific=Any fixed-point  DtypeIntSpecific=Any integer  SampleMode=Ignore
      settings: SourceProductName=DSP System Toolbox  SourceProductBaseCode=DS
  Out1 : Outport
  wires:
  Check Signal Attributes/1 -> Check Signal Attributes1/1
  Check Signal Attributes1/1 -> Out1/1
  In1/1 -> Check Signal Attributes/1

== system Satellte_Communications_System_TDMA/Receiver System Noise Temperature2/Receiver Thermal Noise/Check Input Signal ==
  In1 : Inport
  Check Signal Attributes : dspsigattribs/Check Signal Attributes  SigAttribCheckMethod=Does not match attributes exactly  Complexity=Complex  Frame=Ignore  DimsCheckMethod=Is...  Dimensions=Column vector (2-D) or scalar  DatatypeCheckMethod=Is...  DatatypeGeneral=Floating-point  DtypeFloatSpecific=Any floating-point  DtypeFixedSpecific=Any fixed-point  DtypeIntSpecific=Any integer  SampleMode=Ignore
      settings: SourceProductName=DSP System Toolbox  SourceProductBaseCode=DS
  Check Signal Attributes1 : dspsigattribs/Check Signal Attributes  SigAttribCheckMethod=Matches attributes exactly  Complexity=Ignore  Frame=Sample-based  DimsCheckMethod=Is...  Dimensions=Vector (1-D or 2-D)  DatatypeCheckMethod=Ignore  DatatypeGeneral=Boolean  DtypeFloatSpecific=Any floating-point  DtypeFixedSpecific=Any fixed-point  DtypeIntSpecific=Any integer  SampleMode=Ignore
      settings: SourceProductName=DSP System Toolbox  SourceProductBaseCode=DS
  Out1 : Outport
  wires:
  Check Signal Attributes/1 -> Check Signal Attributes1/1
  Check Signal Attributes1/1 -> Out1/1
  In1/1 -> Check Signal Attributes/1
